simulink model "Set_Speed_Harness"  (R2022b)
settings: configuration reference "CommonModelConfiguration" (kept outside this file)
(part 1 of 3)
settings Model: Creator=AJOSHI11  LastModifiedBy=AJOSHI11
settings ConfigSetRef: SourceName=CommonModelConfiguration  SourceLocation=Base Workspace

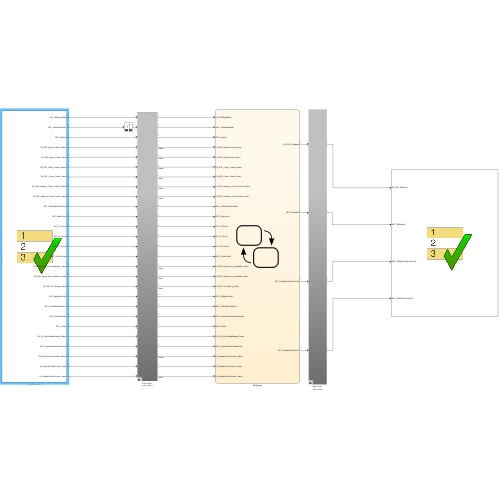
[thumbnail: Simulink's stored preview of the top-level diagram]
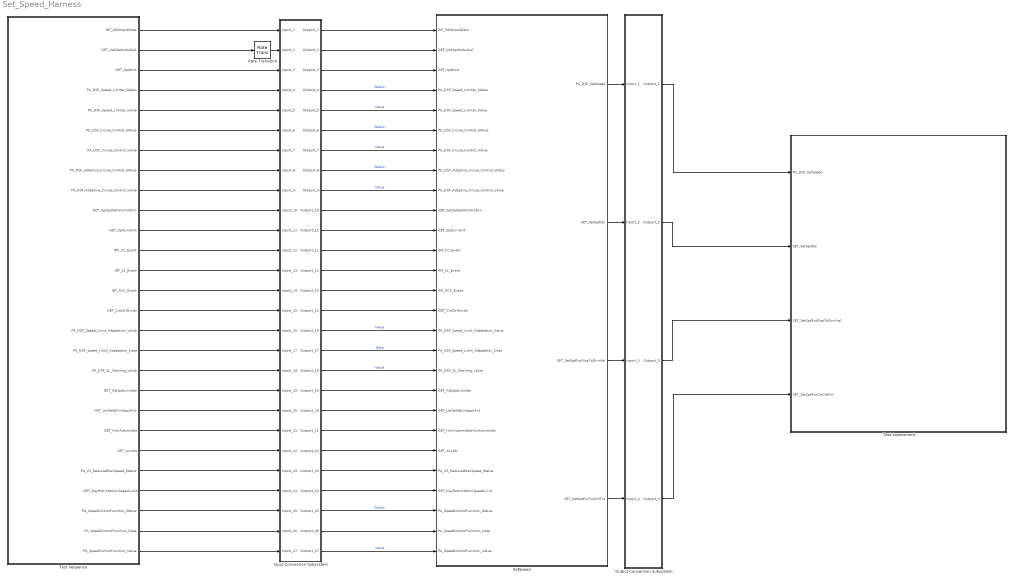
== system Set_Speed_Harness ==
  Input Conversion Subsystem : Subsystem  Tag=__SLT_ICS__  Description=|
      | Signal spec.
      | and routing
      settings: AttributesFormatString=%<Description>
  Output Conversion Subsystem : Subsystem  Tag=__SLT_OCS__  Description=|
      | Signal spec.
      | and routing
      settings: AttributesFormatString=%<Description>
  Rate Transition : RateTransition
  SetSpeed : Stateflow chart  TreatAsAtomicUnit=on
  Test Assessment : Test Sequence  TreatAsAtomicUnit=on
  Test Sequence : Test Sequence  TreatAsAtomicUnit=on
  wires:
  Test Sequence/16(PA_DSF_Speed_Limit_Adaptation_Value) -> Input Conversion Subsystem/16(Inport_16)
  Test Sequence/8(PA_DSF_Adaptive_Cruise_Control_Status) -> Input Conversion Subsystem/8(Inport_8)
  Rate Transition/1 -> Input Conversion Subsystem/2(Inport_2)
  Test Sequence/15(GET_CrsCtrlOvrdn) -> Input Conversion Subsystem/15(Inport_15)
  Test Sequence/7(PA_DSF_Cruise_Control_Value) -> Input Conversion Subsystem/7(Inport_7)
  Test Sequence/14(INT_ACC_Event) -> Input Conversion Subsystem/14(Inport_14)
  Test Sequence/6(PA_DSF_Cruise_Control_Status) -> Input Conversion Subsystem/6(Inport_6)
  Test Sequence/21(GET_HmiAutnmsSts) -> Input Conversion Subsystem/21(Inport_21)
  Test Sequence/13(INT_SL_Event) -> Input Conversion Subsystem/13(Inport_13)
  Test Sequence/5(PA_DSF_Speed_Limiter_Value) -> Input Conversion Subsystem/5(Inport_5)
  Test Sequence/20(GET_UsrSeldDrvrSpprtFct) -> Input Conversion Subsystem/20(Inport_20)
  Test Sequence/12(INT_CC_Event) -> Input Conversion Subsystem/12(Inport_12)
  Test Sequence/4(PA_DSF_Speed_Limiter_Status) -> Input Conversion Subsystem/4(Inport_4)
  Test Sequence/19(GET_AdjSpdLimnSts) -> Input Conversion Subsystem/19(Inport_19)
  Test Sequence/11(GET_SpdLimUnit) -> Input Conversion Subsystem/11(Inport_11)
  Test Sequence/3(GET_SpdUnit) -> Input Conversion Subsystem/3(Inport_3)
  Test Sequence/18(PA_DSF_SL_Warning_Value) -> Input Conversion Subsystem/18(Inport_18)
  Test Sequence/2(GET_VehSpdIndcdVal) -> Rate Transition/1
  Test Sequence/17(PA_DSF_Speed_Limit_Adaptation_Data) -> Input Conversion Subsystem/17(Inport_17)
  Test Sequence/9(PA_DSF_Adaptive_Cruise_Control_Value) -> Input Conversion Subsystem/9(Inport_9)
  Test Sequence/1(INT_SWSInputData) -> Input Conversion Subsystem/1(Inport_1)
  Test Sequence/10(GET_SetSpdSelnForAutDrv) -> Input Conversion Subsystem/10(Inport_10)
  Test Sequence/22(GET_AccSts) -> Input Conversion Subsystem/22(Inport_22)
  Test Sequence/23(PA_VS_ReducedMaxSpeed_Status) -> Input Conversion Subsystem/23(Inport_23)
  Test Sequence/24(GET_KeyRstrictdActvSpeedLimit) -> Input Conversion Subsystem/24(Inport_24)
  Test Sequence/25(PA_SpeedControlFunction_Status) -> Input Conversion Subsystem/25(Inport_25)
  Test Sequence/26(PA_SpeedControlFunction_Data) -> Input Conversion Subsystem/26(Inport_26)
  Test Sequence/27(PA_SpeedControlFunction_Value) -> Input Conversion Subsystem/27(Inport_27)
  Input Conversion Subsystem/9(Outport_9) -> SetSpeed/9(PA_DSF_Adaptive_Cruise_Control_Value)  "Value"
  Input Conversion Subsystem/1(Outport_1) -> SetSpeed/1(INT_SWSInputData)
  Input Conversion Subsystem/10(Outport_10) -> SetSpeed/10(GET_SetSpdSelnForAutDrv)
  Input Conversion Subsystem/2(Outport_2) -> SetSpeed/2(GET_VehSpdIndcdVal)
  Input Conversion Subsystem/11(Outport_11) -> SetSpeed/11(GET_SpdLimUnit)
  Input Conversion Subsystem/3(Outport_3) -> SetSpeed/3(GET_SpdUnit)
  Output Conversion Subsystem/4(Outport_4) -> Test Assessment/4(SET_SetSpdForCrsCtrlFct)
  Input Conversion Subsystem/12(Outport_12) -> SetSpeed/12(INT_CC_Event)
  Input Conversion Subsystem/4(Outport_4) -> SetSpeed/4(PA_DSF_Speed_Limiter_Status)  "Status"
  Input Conversion Subsystem/5(Outport_5) -> SetSpeed/5(PA_DSF_Speed_Limiter_Value)  "Value"
  Input Conversion Subsystem/6(Outport_6) -> SetSpeed/6(PA_DSF_Cruise_Control_Status)  "Status"
  Input Conversion Subsystem/7(Outport_7) -> SetSpeed/7(PA_DSF_Cruise_Control_Value)  "Value"
  Input Conversion Subsystem/8(Outport_8) -> SetSpeed/8(PA_DSF_Adaptive_Cruise_Control_Status)  "Status"
  Input Conversion Subsystem/21(Outport_21) -> SetSpeed/21(GET_HmiAutnmsStsHmiAutnmsSts)
  Input Conversion Subsystem/13(Outport_13) -> SetSpeed/13(INT_SL_Event)
  Input Conversion Subsystem/22(Outport_22) -> SetSpeed/22(GET_AccSts)
  Input Conversion Subsystem/14(Outport_14) -> SetSpeed/14(INT_ACC_Event)
  Input Conversion Subsystem/23(Outport_23) -> SetSpeed/23(PA_VS_ReducedMaxSpeed_Status)
  Input Conversion Subsystem/15(Outport_15) -> SetSpeed/15(GET_CrsCtrlOvrdn)
  Input Conversion Subsystem/24(Outport_24) -> SetSpeed/24(GET_KeyRstrictdActvSpeedLimit)
  Input Conversion Subsystem/16(Outport_16) -> SetSpeed/16(PA_DSF_Speed_Limit_Adaptation_Value)  "Value"
  Input Conversion Subsystem/25(Outport_25) -> SetSpeed/25(PA_SpeedControlFunction_Status)  "Status"
  Input Conversion Subsystem/17(Outport_17) -> SetSpeed/17(PA_DSF_Speed_Limit_Adaptation_Data)  "Data"
  Input Conversion Subsystem/26(Outport_26) -> SetSpeed/26(PA_SpeedControlFunction_Data)
  Input Conversion Subsystem/18(Outport_18) -> SetSpeed/18(PA_DSF_SL_Warning_Value)  "Value"
  Input Conversion Subsystem/27(Outport_27) -> SetSpeed/27(PA_SpeedControlFunction_Value)  "Value"
  Input Conversion Subsystem/19(Outport_19) -> SetSpeed/19(GET_AdjSpdLimnSts)
  Input Conversion Subsystem/20(Outport_20) -> SetSpeed/20(GET_UsrSeldDrvrSpprtFct)
  SetSpeed/1(PA_DSF_SetSpeed) -> Output Conversion Subsystem/1(Inport_1)
  SetSpeed/2(SET_SetSpdSts) -> Output Conversion Subsystem/2(Inport_2)
  SetSpeed/3(SET_SetSpdForDispToDrvrVal) -> Output Conversion Subsystem/3(Inport_3)
  SetSpeed/4(SET_SetSpdForCrsCtrlFct) -> Output Conversion Subsystem/4(Inport_4)
  Output Conversion Subsystem/1(Outport_1) -> Test Assessment/1(PA_DSF_SetSpeed)
  Output Conversion Subsystem/2(Outport_2) -> Test Assessment/2(SET_SetSpdSts)
  Output Conversion Subsystem/3(Outport_3) -> Test Assessment/3(SET_SetSpdForDispToDrvrVal)

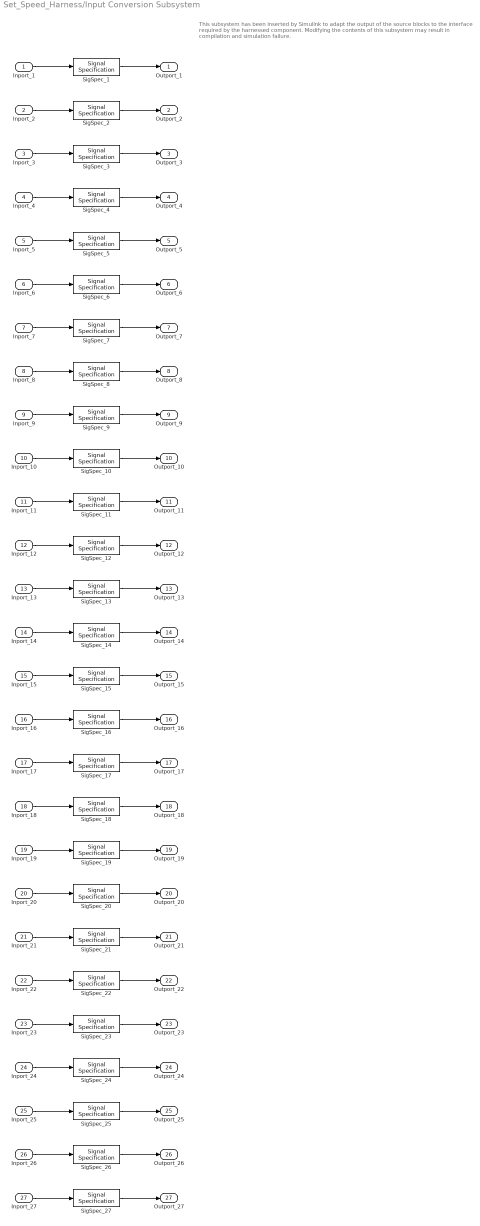
== system Set_Speed_Harness/Input Conversion Subsystem ==
  note: This subsystem has been inserted by Simulink to adapt the output of the source blocks to the interface required by the harnessed component.
      |  Modifying the contents of this subsystem may result in compilation and simulation failure.
  Inport_1 : Inport
  Inport_2 : Inport  Port=2
  Inport_3 : Inport  Port=3
  Inport_4 : Inport  Port=4
  Inport_5 : Inport  Port=5
  Inport_6 : Inport  Port=6
  Inport_7 : Inport  Port=7
  Inport_8 : Inport  Port=8
  Inport_9 : Inport  Port=9
  Inport_10 : Inport  Port=10
  Inport_11 : Inport  Port=11
  Inport_12 : Inport  Port=12
  Inport_13 : Inport  Port=13
  Inport_14 : Inport  Port=14
  Inport_15 : Inport  Port=15
  Inport_16 : Inport  Port=16
  Inport_17 : Inport  Port=17
  Inport_18 : Inport  Port=18
  Inport_19 : Inport  Port=19
  Inport_20 : Inport  Port=20
  Inport_21 : Inport  Port=21
  Inport_22 : Inport  Port=22
  Inport_23 : Inport  Port=23
  Inport_24 : Inport  Port=24
  Inport_25 : Inport  Port=25
  Inport_26 : Inport  Port=26
  Inport_27 : Inport  Port=27
  SigSpec_1 : SignalSpecification  OutDataTypeStr=Bus: SWSInputData  Dimensions=[1]  SampleTime=[0, 0]  BusOutputAsStruct=on
  SigSpec_10 : SignalSpecification  OutDataTypeStr=Enum: SetSpdSelnForAutDrv1  Dimensions=[1]  SampleTime=[0, 0]
  SigSpec_11 : SignalSpecification  OutDataTypeStr=Enum: SpdUnit1  Dimensions=[1]  SampleTime=[0, 0]
  SigSpec_12 : SignalSpecification  OutDataTypeStr=Enum: E_DSF_Event  Dimensions=[1]  SampleTime=[0, 0]
  SigSpec_13 : SignalSpecification  OutDataTypeStr=Enum: E_DSF_Event  Dimensions=[1]  SampleTime=[0, 0]
  SigSpec_14 : SignalSpecification  OutDataTypeStr=Enum: E_DSF_Event  Dimensions=[1]  SampleTime=[0, 0]
  SigSpec_15 : SignalSpecification  OutDataTypeStr=Enum: OnOff1  Dimensions=[1]  SampleTime=[0, 0]
  SigSpec_{5,7,9,16} (4 alike) : SignalSpecification  OutDataTypeStr=Enum: E_DSF_Value  Dimensions=[1]  SampleTime=[0, 0]
  SigSpec_{2,17,24,26} (4 alike) : SignalSpecification  OutDataTypeStr=double  Dimensions=[1]  SampleTime=[0, 0]
  SigSpec_18 : SignalSpecification  OutDataTypeStr=Enum: E_OffOn  Dimensions=[1]  SampleTime=[0, 0]
  SigSpec_19 : SignalSpecification  OutDataTypeStr=Enum: AdjSpdLimnSts2  Dimensions=[1]  SampleTime=[0, 0]
  SigSpec_20 : SignalSpecification  OutDataTypeStr=Enum: DrvrSpprtFct  Dimensions=[1]  SampleTime=[0, 0]
  SigSpec_21 : SignalSpecification  OutDataTypeStr=Enum: HmiAutnmsSts1  Dimensions=[1]  SampleTime=[0, 0]
  SigSpec_22 : SignalSpecification  OutDataTypeStr=Enum: AccSts1  Dimensions=[1]  SampleTime=[0, 0]
  SigSpec_{4,6,8,23,25} (5 alike) : SignalSpecification  OutDataTypeStr=Enum: E_CommonStatus  Dimensions=[1]  SampleTime=[0, 0]
  SigSpec_27 : SignalSpecification  OutDataTypeStr=Enum: E_OffOn  Dimensions=[1]  SampleTime=[0, 0]
  SigSpec_3 : SignalSpecification  OutDataTypeStr=Enum: VehSpdIndcdUnit  Dimensions=[1]  SampleTime=[0, 0]
  Outport_1 : Outport
  Outport_2 : Outport  Port=2
  Outport_3 : Outport  Port=3
  Outport_4 : Outport  Port=4
  Outport_5 : Outport  Port=5
  Outport_6 : Outport  Port=6
  Outport_7 : Outport  Port=7
  Outport_8 : Outport  Port=8
  Outport_9 : Outport  Port=9
  Outport_10 : Outport  Port=10
  Outport_11 : Outport  Port=11
  Outport_12 : Outport  Port=12
  Outport_13 : Outport  Port=13
  Outport_14 : Outport  Port=14
  Outport_15 : Outport  Port=15
  Outport_16 : Outport  Port=16
  Outport_17 : Outport  Port=17
  Outport_18 : Outport  Port=18
  Outport_19 : Outport  Port=19
  Outport_20 : Outport  Port=20
  Outport_21 : Outport  Port=21
  Outport_22 : Outport  Port=22
  Outport_23 : Outport  Port=23
  Outport_24 : Outport  Port=24
  Outport_25 : Outport  Port=25
  Outport_26 : Outport  Port=26
  Outport_27 : Outport  Port=27
  wires:
  SigSpec_1/1 -> Outport_1/1
  Inport_1/1 -> SigSpec_1/1
  SigSpec_2/1 -> Outport_2/1
  Inport_2/1 -> SigSpec_2/1
  SigSpec_3/1 -> Outport_3/1
  Inport_3/1 -> SigSpec_3/1
  SigSpec_4/1 -> Outport_4/1
  Inport_4/1 -> SigSpec_4/1
  SigSpec_5/1 -> Outport_5/1
  Inport_5/1 -> SigSpec_5/1
  SigSpec_6/1 -> Outport_6/1
  Inport_6/1 -> SigSpec_6/1
  SigSpec_7/1 -> Outport_7/1
  Inport_7/1 -> SigSpec_7/1
  SigSpec_8/1 -> Outport_8/1
  Inport_8/1 -> SigSpec_8/1
  SigSpec_9/1 -> Outport_9/1
  Inport_9/1 -> SigSpec_9/1
  SigSpec_10/1 -> Outport_10/1
  Inport_10/1 -> SigSpec_10/1
  SigSpec_11/1 -> Outport_11/1
  Inport_11/1 -> SigSpec_11/1
  SigSpec_12/1 -> Outport_12/1
  Inport_12/1 -> SigSpec_12/1
  SigSpec_13/1 -> Outport_13/1
  Inport_13/1 -> SigSpec_13/1
  SigSpec_14/1 -> Outport_14/1
  Inport_14/1 -> SigSpec_14/1
  SigSpec_15/1 -> Outport_15/1
  Inport_15/1 -> SigSpec_15/1
  SigSpec_16/1 -> Outport_16/1
  Inport_16/1 -> SigSpec_16/1
  SigSpec_17/1 -> Outport_17/1
  Inport_17/1 -> SigSpec_17/1
  SigSpec_18/1 -> Outport_18/1
  Inport_18/1 -> SigSpec_18/1
  SigSpec_19/1 -> Outport_19/1
  Inport_19/1 -> SigSpec_19/1
  SigSpec_20/1 -> Outport_20/1
  Inport_20/1 -> SigSpec_20/1
  SigSpec_21/1 -> Outport_21/1
  Inport_21/1 -> SigSpec_21/1
  SigSpec_22/1 -> Outport_22/1
  Inport_22/1 -> SigSpec_22/1
  SigSpec_23/1 -> Outport_23/1
  Inport_23/1 -> SigSpec_23/1
  SigSpec_24/1 -> Outport_24/1
  Inport_24/1 -> SigSpec_24/1
  SigSpec_25/1 -> Outport_25/1
  Inport_25/1 -> SigSpec_25/1
  SigSpec_26/1 -> Outport_26/1
  Inport_26/1 -> SigSpec_26/1
  SigSpec_27/1 -> Outport_27/1
  Inport_27/1 -> SigSpec_27/1

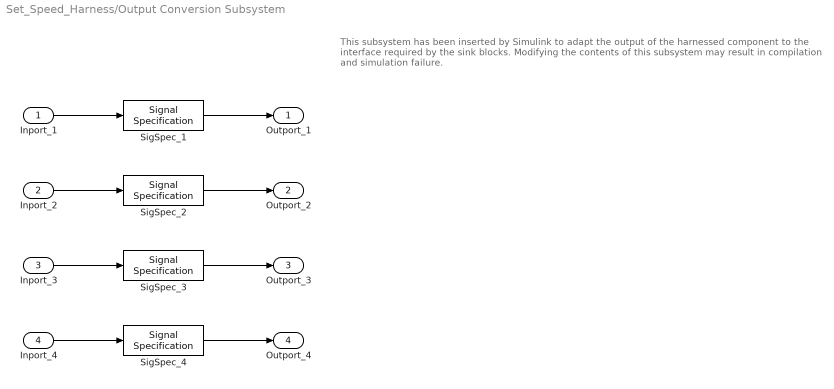
== system Set_Speed_Harness/Output Conversion Subsystem ==
  note: This subsystem has been inserted by Simulink to adapt the output of the harnessed component to the interface required by the sink blocks.
      |  Modifying the contents of this subsystem may result in compilation and simulation failure.
  Inport_1 : Inport
  Inport_2 : Inport  Port=2
  Inport_3 : Inport  Port=3
  Inport_4 : Inport  Port=4
  SigSpec_1 : SignalSpecification  OutDataTypeStr=Bus: PA_StatusAndValueAndDoubleAndDouble  Dimensions=[1]  BusOutputAsStruct=on
  SigSpec_2 : SignalSpecification  OutDataTypeStr=Enum: SetSpdSts1  Dimensions=[1]
  SigSpec_3 : SignalSpecification  OutDataTypeStr=double  Dimensions=[1]
  SigSpec_4 : SignalSpecification  OutDataTypeStr=double  Dimensions=[1]
  Outport_1 : Outport
  Outport_2 : Outport  Port=2
  Outport_3 : Outport  Port=3
  Outport_4 : Outport  Port=4
  wires:
  Inport_1/1 -> SigSpec_1/1
  SigSpec_1/1 -> Outport_1/1
  Inport_2/1 -> SigSpec_2/1
  SigSpec_2/1 -> Outport_2/1
  Inport_3/1 -> SigSpec_3/1
  SigSpec_3/1 -> Outport_3/1
  Inport_4/1 -> SigSpec_4/1
  SigSpec_4/1 -> Outport_4/1

== stateflow chart Set_Speed_Harness/Test Assessment ==
  state step_1
    state step_1_1
    state step_1_2
      verify(abs(PA_DSF_SetSpeed.SetSpeed) < 1e-6);
      verify(PA_DSF_SetSpeed.Status == E_CommonStatus.Disabled);
      verify(PA_DSF_SetSpeed.Value == E_DSF_Value.DSF_Off);
    step_1 -> (junction 70) [order 1]
    (default) -> (junction 70)
    (junction 80) -> step_1_1 [order 1] : [~in(step_1.step_1_1)]
    (junction 70) -> (junction 80) [order 1] : [t>1
        | ]
    (junction 80) -> (junction 83) [order 2]
    (junction 91) -> (junction 92)
    (junction 92) -> step_1_2 [order 1] : [~in(step_1.step_1_2)]
    (junction 92) -> (junction 95) [order 2]
    (junction 70) -> (junction 91) [order 2]
  state step_2
    verify(abs(PA_DSF_SetSpeed.SetSpeed - 70) <= 1e-3);
    verify(PA_DSF_SetSpeed.Status == E_CommonStatus.Available);
    verify(PA_DSF_SetSpeed.Value == E_DSF_Value.DSF_Overridden);
  state step_3
    verify(PA_DSF_SetSpeed.Status == E_CommonStatus.Available);
  (default) -> step_1
  step_1 -> step_2 [order 1] : [
      | after(3.1,sec)
      | ]
  step_2 -> step_3
  data: PA_DSF_SetSpeed input; SET_SetSpdSts input; SET_SetSpdForDispToDrvrVal input; SET_SetSpdForCrsCtrlFct input
